simulink model "project"  (R2020a)
settings: Solver=VariableStepAuto  StartTime=0.0  StopTime=1000  RelTol=1e-3
values from neighbouring files (symbols this model uses):
  a = (6371+h)*1e3    (= 6871000)    [AMM_main.m]    (also in Data.m)
  A_RW = sqrt([prop1;prop2;prop3]/(prop1+prop2+prop3))    [AMM_main.m]    (also in Data.m)
  A_t = [Ax;Ay;Az;Ax;Ay;Az;A_sp;A_sp;A_sp;A_sp;]    [AMM_main.m]    (also in Data.m)
  alpha = 0.005    [AMM_main.m]    (also in Data.m = 0.5)
  cd = 2.2    [AMM_main.m]    (also in Data.m)
  horiz_ang_err = rand(3,1) - 0.5    [Data.m]
  horiz_err = 0.25*pi/180    (= 0.00436332312999)    [Data.m]
  init_DCM = DCM0_track    [AMM_main.m]    (also in Data.m = [0.097540404999410   0.957506835434298   0.970592781760616)
  init_orb = orb0_track    [AMM_main.m]    (also in Data.m = [e0,i0,O0,o0,th0])
  init_tumbl = w0_track    [AMM_main.m]    (also in Data.m = 10*pi/180*dir)
  Ir = 1e-7    (= 1e-07)    [AMM_main.m]    (also in Data.m)
  Iz = 2e-7    (= 2e-07)    [AMM_main.m]    (also in Data.m)
  J = [Jx;Jy;Jz]    [AMM_main.m]    (also in Data.m)
  K1 = .05    (= 0.05)    [AMM_main.m]    (also in Data.m)
  K2 = 0.5*K1^2    (= 0.00125)    [AMM_main.m]    (also in Data.m)
  magn_ang_err = rand(3,1) - 0.5    [Data.m]
  magn_err = 2*pi/180    (= 0.0349065850399)    [Data.m]
  max_mx = 1.19    [AMM_main.m]    (also in Data.m)
  max_my = 1.19    [AMM_main.m]    (also in Data.m)
  max_mz = 1.19    [AMM_main.m]    (also in Data.m)
  MS_freq = 1    [AMM_main.m]    (also in Data.m)
  mu = 3.986004418e14    (= 398600441800000)    [AMM_main.m]    (also in Data.m)
  n = sqrt( mu / a^3 )    [AMM_main.m]    (also in Data.m)
  rho = [rho_sMB;rho_dMB;rho_sSP;rho_dSP]    [AMM_main.m]    (also in Data.m)
  rho_air = 4.39e-16 * 1e6/1e3    (= 4.39e-13)    [AMM_main.m]    (also in Data.m)
  RW_Ir = 3.4e-4    (= 0.00034)    [AMM_main.m]    (also in Data.m)
  RW_max_momentum = 400e-3    (= 0.4)    [AMM_main.m]    (also in Data.m)
  RW_max_torque = 100e-3    (= 0.1)    [AMM_main.m]    (also in Data.m)
  wr = 100*pi/180    (= 1.74532925199)    [AMM_main.m]    (also in Data.m)
  ww_earth = 2*pi/(24*3600)*[0;0;1]    [AMM_main.m]    (also in Data.m)
libraries: vrlib x6, simulink x5, dspmtrx3 x2
(part 2 of 2)

== matlab function project/reference DCM/s//c position for a given orbit/Earth's position ==
  data: a input; orb_elements input; r_N output; v_N output
function [r_N,v_N]  = Earth_pos(a,orb_elements)

mu = 3.986004418e14;

e_mod = orb_elements(1);
i     = orb_elements(2);
Omega = orb_elements(3);
omega = orb_elements(4);
theta = orb_elements(5);


h_mod = sqrt(mu*a*(1-e_mod^2));
    
e_unit = rotation_matrix_R3(-Omega) * ...
         rotation_matrix_R1(-i) * ...
         rotation_matrix_R3(-omega) * [1;0;0];
p_unit = rotation_matrix_R3(-Omega) * ...
         rotation_matrix_R1(-i) * ...
         rotation_matrix_R3(-omega) * [0;1;0];
     
r_mod_0 = h_mod^2/mu/(1+e_mod*cos(theta));
r_N       = r_mod_0 * ( cos(theta) * e_unit  +  sin(theta) * p_unit );
v_r     = mu/h_mod * e_mod*sin(theta);
v_theta = mu/h_mod * (1 + e_mod*cos(theta));
v_N       = v_r     * (  cos(theta) * e_unit  +  sin(theta) * p_unit )+ ...
          v_theta * ( -sin(theta) * e_unit  +  cos(theta) * p_unit );
end


function R1 = rotation_matrix_R1(alpha)
%{
rotation_matrix_R1: computes rotation matrix of angle alpha around x axis

INPUT:
	alpha[1]                Angle rotated
                                [rad]

OUTPUT:
    R1 [3x3]                Rotation matrix
                                [(3x3) x -]
%}

R1 = zeros(3);

R1(1,1) = 1;
R1(2,2) =  cos(alpha);
R1(2,3) =  sin(alpha);
R1(3,2) = -sin(alpha);
R1(3,3) =  cos(alpha);
end


function R3 = rotation_matrix_R3(alpha)
%{
rotation_matrix_R3: computes rotation matrix of angle alpha around z axis

INPUT:
	alpha[1]                Angle rotated
                                [rad]

OUTPUT:
    R3 [3x3]                Rotation matrix
                                [(3x3) x -]

%}

R3 = zeros(3);

R3(1,1) =  cos(alpha);
R3(1,2) =  sin(alpha);
R3(2,1) = -sin(alpha);
R3(2,2) =  cos(alpha);
R3(3,3) =  1;
end

== matlab function project/reference DCM/s//c position for a given orbit/orb_elements dynamics/sat motion ==
  data: a input; orb_elements input; orb_elements_dot output
function orb_elements_dot = orbit(a,orb_elements)

mu = 3.986004418e14;

e     = orb_elements(1);
i     = orb_elements(2);
O = orb_elements(3);
o = orb_elements(4);
theta = orb_elements(5); %true anomaly


n     = sqrt( mu / a^3 ); %mean motion: angular speed required to complete 1 orbit

orb_elements_dot    = zeros (size(orb_elements));

orb_elements_dot(5) = n * (1 + e*cos(theta))^2 / (1 - e^2)^(3/2);

== matlab function project/Sun direction wrt s//c body frame/Sun's direction ==
  data: t input; S_N output
function S_N = fcn(t)

%% data
Rs = 149597870700; %[m] but we can substitute it by 1 so we have a unitary vector
Rs = 1;
epsilon = 23.45 * pi/180; %[rad]
T = 365.25*24*3600; %[s]
nsun = 2*pi/T; % [s^-1]

%% 
S_N = Rs * [cos(nsun*t);
            sin(nsun*t)*cos(epsilon);
            sin(nsun*t)*sin(epsilon);];

end

== matlab function project/magnetic torquer detumbling control/magn.vector body frame/Magnetic model ==
  data: r_N input; b_N output; t input
function b_N = fcn(r_N,t)
% coefficients
IGRF = '2000';
switch IGRF
    case '1995'
        g0_1 = -29682e-9;
        g1_1 = -1789e-9;
        h1_1 = 5318e-9;
    case '2000'
        g0_1 = -29615e-9;
        g1_1 = -1728e-9;
        h1_1 = 5186e-9;
end


w = 360/(24*3600) * pi/180; %[rad/s] angular rotation speed of Earth
decl = 11.5*pi/180; %[rad]
R = 6371.2e3; %equatorial radius [m]
r = norm(r_N);
rr_unit = r_N/r; %unitary vector

H0 = sqrt(g0_1^2 + g1_1^2 + h1_1^2);
m = [
    sin(decl)*cos(w*t);
    sin(decl)*sin(w*t);
    cos(decl)
    ]; %unit vector along dipole axis

b_N = R^3*H0/r^3*(3*(dot(m,rr_unit))*rr_unit - m); %Earth's MF in the inertial frame

== matlab function project/magnetic torquer detumbling control/magn.vector body frame/s//c position for a given orbit/Earth's position ==
  data: a input; orb_elements input; r_N output; v_N output
function [r_N,v_N]  = Earth_pos(a,orb_elements)

mu = 3.986004418e14;

e_mod = orb_elements(1);
i     = orb_elements(2);
Omega = orb_elements(3);
omega = orb_elements(4);
theta = orb_elements(5);


h_mod = sqrt(mu*a*(1-e_mod^2));
    
e_unit = rotation_matrix_R3(-Omega) * ...
         rotation_matrix_R1(-i) * ...
         rotation_matrix_R3(-omega) * [1;0;0];
p_unit = rotation_matrix_R3(-Omega) * ...
         rotation_matrix_R1(-i) * ...
         rotation_matrix_R3(-omega) * [0;1;0];
     
r_mod_0 = h_mod^2/mu/(1+e_mod*cos(theta));
r_N       = r_mod_0 * ( cos(theta) * e_unit  +  sin(theta) * p_unit );
v_r     = mu/h_mod * e_mod*sin(theta);
v_theta = mu/h_mod * (1 + e_mod*cos(theta));
v_N       = v_r     * (  cos(theta) * e_unit  +  sin(theta) * p_unit )+ ...
          v_theta * ( -sin(theta) * e_unit  +  cos(theta) * p_unit );
end


function R1 = rotation_matrix_R1(alpha)
%{
rotation_matrix_R1: computes rotation matrix of angle alpha around x axis

INPUT:
	alpha[1]                Angle rotated
                                [rad]

OUTPUT:
    R1 [3x3]                Rotation matrix
                                [(3x3) x -]
%}

R1 = zeros(3);

R1(1,1) = 1;
R1(2,2) =  cos(alpha);
R1(2,3) =  sin(alpha);
R1(3,2) = -sin(alpha);
R1(3,3) =  cos(alpha);
end


function R3 = rotation_matrix_R3(alpha)
%{
rotation_matrix_R3: computes rotation matrix of angle alpha around z axis

INPUT:
	alpha[1]                Angle rotated
                                [rad]

OUTPUT:
    R3 [3x3]                Rotation matrix
                                [(3x3) x -]

%}

R3 = zeros(3);

R3(1,1) =  cos(alpha);
R3(1,2) =  sin(alpha);
R3(2,1) = -sin(alpha);
R3(2,2) =  cos(alpha);
R3(3,3) =  1;
end

== matlab function project/Disturbances: -grav.gradient -airdrag -SRP -magnetic field/magnetic torque/magnetic model/Magnetic model ==
  data: r_N input; b_N output; t input
function b_N = fcn(r_N,t)
% coefficients
IGRF = '2000';
switch IGRF
    case '1995'
        g0_1 = -29682e-9;
        g1_1 = -1789e-9;
        h1_1 = 5318e-9;
    case '2000'
        g0_1 = -29615e-9;
        g1_1 = -1728e-9;
        h1_1 = 5186e-9;
end


w = 360/(24*3600) * pi/180; %[rad/s] angular rotation speed of Earth
decl = 11.5*pi/180; %[rad]
R = 6371.2e3; %equatorial radius [m]
r = norm(r_N);
rr_unit = r_N/r; %unitary vector

H0 = sqrt(g0_1^2 + g1_1^2 + h1_1^2);
m = [
    sin(decl)*cos(w*t);
    sin(decl)*sin(w*t);
    cos(decl)
    ]; %unit vector along dipole axis

b_N = R^3*H0/r^3*(3*(dot(m,rr_unit))*rr_unit - m); %Earth's MF in the inertial frame

== matlab function project/Disturbances: -grav.gradient -airdrag -SRP -magnetic field/magnetic torque/magnetic model/s//c position for a given orbit/Earth's position ==
  data: a input; orb_elements input; r_N output; v_N output
function [r_N,v_N]  = Earth_pos(a,orb_elements)

mu = 3.986004418e14;

e_mod = orb_elements(1);
i     = orb_elements(2);
Omega = orb_elements(3);
omega = orb_elements(4);
theta = orb_elements(5);


h_mod = sqrt(mu*a*(1-e_mod^2));
    
e_unit = rotation_matrix_R3(-Omega) * ...
         rotation_matrix_R1(-i) * ...
         rotation_matrix_R3(-omega) * [1;0;0];
p_unit = rotation_matrix_R3(-Omega) * ...
         rotation_matrix_R1(-i) * ...
         rotation_matrix_R3(-omega) * [0;1;0];
     
r_mod_0 = h_mod^2/mu/(1+e_mod*cos(theta));
r_N       = r_mod_0 * ( cos(theta) * e_unit  +  sin(theta) * p_unit );
v_r     = mu/h_mod * e_mod*sin(theta);
v_theta = mu/h_mod * (1 + e_mod*cos(theta));
v_N       = v_r     * (  cos(theta) * e_unit  +  sin(theta) * p_unit )+ ...
          v_theta * ( -sin(theta) * e_unit  +  cos(theta) * p_unit );
end


function R1 = rotation_matrix_R1(alpha)
%{
rotation_matrix_R1: computes rotation matrix of angle alpha around x axis

INPUT:
	alpha[1]                Angle rotated
                                [rad]

OUTPUT:
    R1 [3x3]                Rotation matrix
                                [(3x3) x -]
%}

R1 = zeros(3);

R1(1,1) = 1;
R1(2,2) =  cos(alpha);
R1(2,3) =  sin(alpha);
R1(3,2) = -sin(alpha);
R1(3,3) =  cos(alpha);
end


function R3 = rotation_matrix_R3(alpha)
%{
rotation_matrix_R3: computes rotation matrix of angle alpha around z axis

INPUT:
	alpha[1]                Angle rotated
                                [rad]

OUTPUT:
    R3 [3x3]                Rotation matrix
                                [(3x3) x -]

%}

R3 = zeros(3);

R3(1,1) =  cos(alpha);
R3(1,2) =  sin(alpha);
R3(2,1) = -sin(alpha);
R3(2,2) =  cos(alpha);
R3(3,3) =  1;
end

== matlab function project/Disturbances: -grav.gradient -airdrag -SRP -magnetic field/magnetic torque/magnetic model/s//c position for a given orbit/orb_elements dynamics/sat motion ==
  data: a input; orb_elements input; orb_elements_dot output
function orb_elements_dot = orbit(a,orb_elements)

mu = 3.986004418e14;

e     = orb_elements(1);
i     = orb_elements(2);
O = orb_elements(3);
o = orb_elements(4);
theta = orb_elements(5); %true anomaly


n     = sqrt( mu / a^3 ); %mean motion: angular speed required to complete 1 orbit

orb_elements_dot    = zeros (size(orb_elements));

orb_elements_dot(5) = n * (1 + e*cos(theta))^2 / (1 - e^2)^(3/2);

== matlab function project/DCM Kinematics/hat ==
  data: w input; w_hat output
function w_hat = hat_fcn(w)

w_hat       = zeros (3);

w_hat (1,2) = - w(3);
w_hat (1,3) =   w(2);
w_hat (2,1) =   w(3);
w_hat (2,3) = - w(1);
w_hat (3,1) = - w(2);
w_hat (3,2) =   w(1);

== matlab function project/magnetic torquer detumbling control/magn.vector body frame/s//c position for a given orbit/orb_elements dynamics/sat motion ==
  data: a input; orb_elements input; orb_elements_dot output
function orb_elements_dot = orbit(a,orb_elements)

mu = 3.986004418e14;

e     = orb_elements(1);
i     = orb_elements(2);
O = orb_elements(3);
o = orb_elements(4);
theta = orb_elements(5); %true anomaly


n     = sqrt( mu / a^3 ); %mean motion: angular speed required to complete 1 orbit

orb_elements_dot    = zeros (size(orb_elements));

orb_elements_dot(5) = n * (1 + e*cos(theta))^2 / (1 - e^2)^(3/2);

== matlab function project/dynamic equation ==
  data: M input; u input; J input; w input; wdot output
function wdot = fcn(M,u,J,w)
%data
% J1 = 100.9e-2; %[kg m^2]
% J2 =  25.1e-2;
% J3 =  91.6e-2;
J1 = J(1);
J2 = J(2);
J3 = J(3);

% diff equation
wdot = zeros(size(w));

wdot(1) = (J2 - J3)/J1 * w(2) * w(3) + u(1)/J1 + M(1)/J1;
wdot(2) = (J3 - J1)/J2 * w(1) * w(3) + u(2)/J2 + M(2)/J2;
wdot(3) = (J1 - J2)/J3 * w(1) * w(2) + u(3)/J3 + M(3)/J3;

end

== matlab function project/Disturbances: -grav.gradient -airdrag -SRP -magnetic field/SRP moment/SRP disturbance torque ==
  data: S_B input; T_srp output; A input; rho input
function T_srp = fcn(S_B,A,rho)

% Solar Radiation Pressure
F_e = 1358;
c   = 3e8;
P   =  F_e / c;

% Displaced CoM
r_CoM = 1.8e-2 * [1; 0; 0]; %considering x-axis displaced

% SC main body
n = zeros(3,10);
n(:,1) = [1; 0; 0];
n(:,2) = [0; 1; 0];
n(:,3) = [0; 0; 1];
n(:,4) = - n(:,1);
n(:,5) = - n(:,2);
n(:,6) = - n(:,3);

% % Area
% A = zeros(10,1);
% A(1) = 6*0.1*0.1; %s/c area
% A(2) = 4*0.1*0.1;
% A(3) = A(1);
% A(4) = A(1);
% A(5) = A(2);
% A(6) = A(3);
% A(7)  = 5*0.1*0.1; %solar panel area
% A(8)  = A(7);
% A(9)  = A(7);
% A(10) = A(9);

% position of center of pressure of the flat surface wrt the center of mass
r = zeros(3,10);
r(:,1) =  0.1*[1; 0; 0] - r_CoM; %typical CoP locations
r(:,2) = 0.15*[0; 1; 0] - r_CoM; %typical CoP locations
r(:,3) =  0.1*[0; 0; 1] - r_CoM; %typical CoP locations
r(:,4) = - r(:,1) - r_CoM;
r(:,5) = - r(:,2) - r_CoM;
r(:,6) = - r(:,3) - r_CoM;

rho_sMB = rho(1);
rho_dMB = rho(2);

% SC solar panels
n(:,7)  =   n(:,1);
n(:,8)  = - n(:,1);
n(:,9)  =   n(:,2);
n(:,10) = - n(:,2);

r(:,7)  =  0.25*[0; 0; 1] - r_CoM;
r(:,8)  =  r(:,7);
r(:,9)  = -0.25*[0; 0; 1] - r_CoM;
r(:,10) =  r(:,9);

rho_sSP = rho(3);
rho_dSP = rho(4);

% Forces on each side and resulting torque
F = zeros(3,10);
for i = 1:6
    if dot(S_B,n(:,i)) > 0
        F(:,i) = - P * A(i) * dot(S_B,n(:,i)) * ...
           (  (1-rho_sMB)*S_B +         ...
             ( 2*rho_sMB*dot(S_B,n(:,i)) + 2/3*rho_dMB) * n(:,i) );
    else
        F(:,i) = [0;0;0];
    end
end

for i = 7:10
    if dot(S_B,n(:,i)) > 0
        F(:,i) = - P * A(i) * dot(S_B,n(:,i)) * ...
           (  (1-rho_sSP)*S_B +         ...
             ( 2*rho_sSP*dot(S_B,n(:,i)) + 2/3*rho_dSP) * n(:,i) );
    else
        F(:,i) = [0;0;0];
    end
end

T_srp = zeros(3,1);
for i=length(F)
    T_srp = T_srp + cross(r(:,i),F(:,i));
end

end %function

== matlab function project/Disturbances: -grav.gradient -airdrag -SRP -magnetic field/air drag/air drag ==
  data: vv_r input; M_drag output; A input; rho input; cd input
function M_drag = fcn(vv_r,A,rho,cd)

v_r = norm(vv_r); % 
% rho = 4.39e-16 * 1e6/1e3; %[kg/m3] rho density at constant altitude 500km
% cd = 2.2; %typical value

% Displaced CoM
r_CoM = 1.8e-2 * [1; 0; 0]; %considering x-axis displaced

% SC main body
n = zeros(3,10);
n(:,1) = [1; 0; 0];
n(:,2) = [0; 1; 0];
n(:,3) = [0; 0; 1];
n(:,4) = - n(:,1);
n(:,5) = - n(:,2);
n(:,6) = - n(:,3);
% SC solar panels
n(:,7)  =   n(:,1);
n(:,8)  = - n(:,1);
n(:,9)  =   n(:,2);
n(:,10) = - n(:,2);

% Area
% A = zeros(10,1);
% A(1) = 6*0.1*0.1;
% A(2) = 4*0.1*0.1;
% A(3) = A(1);
% A(4) = A(1);
% A(5) = A(2);
% A(6) = A(3);
% A(7)  = 5*0.1*0.1;
% A(8)  = A(7);
% A(9)  = A(7);
% A(10) = A(9);

% r: position vector from s/c CoM to CoP of surface Ai
r = zeros(3,10);
r(:,1) =  0.1*[1; 0; 0] - r_CoM; %typical CoP locations
r(:,2) = 0.15*[0; 1; 0] - r_CoM; %typical CoP locations
r(:,3) =  0.1*[0; 0; 1] - r_CoM; %typical CoP locations
r(:,4) = - r(:,1) - r_CoM;
r(:,5) = - r(:,2) - r_CoM;
r(:,6) = - r(:,3) - r_CoM;
r(:,7)  =  0.25*[0; 0; 1] - r_CoM;
r(:,8)  =  r(:,7);
r(:,9)  = -0.25*[0; 0; 1] - r_CoM;
r(:,10) =  r(:,9);

F = zeros(3,10);
M_drag = zeros(3,1);
for i=1:10
    if dot(n(:,i),vv_r/v_r) > 0
        F(:,i) = -0.5*cd*rho*v_r^2*A(i)*vv_r/v_r*dot(n(:,i),vv_r/v_r);
    end
    M_drag = M_drag + cross(r(:,i),F(:,i));
end

end %function

== matlab function project/Disturbances: -grav.gradient -airdrag -SRP -magnetic field/air drag/s//c position for a given orbit/Earth's position ==
  data: a input; orb_elements input; r_N output; v_N output
function [r_N,v_N]  = Earth_pos(a,orb_elements)

mu = 3.986004418e14;

e_mod = orb_elements(1);
i     = orb_elements(2);
Omega = orb_elements(3);
omega = orb_elements(4);
theta = orb_elements(5);


h_mod = sqrt(mu*a*(1-e_mod^2));
    
e_unit = rotation_matrix_R3(-Omega) * ...
         rotation_matrix_R1(-i) * ...
         rotation_matrix_R3(-omega) * [1;0;0];
p_unit = rotation_matrix_R3(-Omega) * ...
         rotation_matrix_R1(-i) * ...
         rotation_matrix_R3(-omega) * [0;1;0];
     
r_mod_0 = h_mod^2/mu/(1+e_mod*cos(theta));
r_N       = r_mod_0 * ( cos(theta) * e_unit  +  sin(theta) * p_unit );
v_r     = mu/h_mod * e_mod*sin(theta);
v_theta = mu/h_mod * (1 + e_mod*cos(theta));
v_N       = v_r     * (  cos(theta) * e_unit  +  sin(theta) * p_unit )+ ...
          v_theta * ( -sin(theta) * e_unit  +  cos(theta) * p_unit );
end


function R1 = rotation_matrix_R1(alpha)
%{
rotation_matrix_R1: computes rotation matrix of angle alpha around x axis

INPUT:
	alpha[1]                Angle rotated
                                [rad]

OUTPUT:
    R1 [3x3]                Rotation matrix
                                [(3x3) x -]
%}

R1 = zeros(3);

R1(1,1) = 1;
R1(2,2) =  cos(alpha);
R1(2,3) =  sin(alpha);
R1(3,2) = -sin(alpha);
R1(3,3) =  cos(alpha);
end


function R3 = rotation_matrix_R3(alpha)
%{
rotation_matrix_R3: computes rotation matrix of angle alpha around z axis

INPUT:
	alpha[1]                Angle rotated
                                [rad]

OUTPUT:
    R3 [3x3]                Rotation matrix
                                [(3x3) x -]

%}

R3 = zeros(3);

R3(1,1) =  cos(alpha);
R3(1,2) =  sin(alpha);
R3(2,1) = -sin(alpha);
R3(2,2) =  cos(alpha);
R3(3,3) =  1;
end

== matlab function project/Disturbances: -grav.gradient -airdrag -SRP -magnetic field/air drag/s//c position for a given orbit/orb_elements dynamics/sat motion ==
  data: a input; orb_elements input; orb_elements_dot output
function orb_elements_dot = orbit(a,orb_elements)

mu = 3.986004418e14;

e     = orb_elements(1);
i     = orb_elements(2);
O = orb_elements(3);
o = orb_elements(4);
theta = orb_elements(5); %true anomaly


n     = sqrt( mu / a^3 ); %mean motion: angular speed required to complete 1 orbit

orb_elements_dot    = zeros (size(orb_elements));

orb_elements_dot(5) = n * (1 + e*cos(theta))^2 / (1 - e^2)^(3/2);

== matlab function project/DCM feedback control/DCM feedback ==
  data: w input; A_e input; K1 input; K2 input; u output; J input; mu input; a input
function u = DCM_fbk_control(w,A_e,K1,K2,J,mu,a)


w_ref = [0; 0; -sqrt(mu/a^3) ];
I_x = J(1);
I_y = J(2);
I_z = J(3);

% u = -K1*w - K2*[A_e(2,3)-A_e(3,2); A_e(3,1)-A_e(1,3); A_e(1,2)-A_e(2,1)];
u = - K1 * [I_x;I_y;I_z].*(w - w_ref) ...
    - K2 * [I_x;I_y;I_z].*[A_e(2,3)-A_e(3,2); A_e(3,1)-A_e(1,3); A_e(1,2)-A_e(2,1)] ...
    + cross ( w, [I_x;I_y;I_z].*w );
%     - K3 * sign(w) ...
%     + K2 * ( (trace(A_e)-1)*[A_e(3,2)-A_e(2,3); A_e(1,3)-A_e(3,1); A_e(2,1)-A_e(1,2)] - w ) ...

% Avoid excesive rotational rate problematic for attitude acquisition (0.5 deg/s)
u_sat_max = - K1 * [I_x;I_y;I_z].*(w - 0.45*pi/180*[1;1;1]/sqrt(3)) ...
            + cross ( w, [I_x;I_y;I_z].*w );
u_sat_min = - K1 * [I_x;I_y;I_z].*(w + 0.45*pi/180*[1;1;1]/sqrt(3)) ...
            + cross ( w, [I_x;I_y;I_z].*w );
for i = 1:3
    if ( u(i)*w(i) > 0 ) && ( abs(w(i)) > 0.4*pi/180/sqrt(3) )
%         u(i) = - K1*w(i);
%         u(i) = - K1*sign(w(i))*(abs(w(i)) - 0.45*pi/180);
        if w(i)>0
            u(i) = u_sat_max(i);
        else
            u(i) = u_sat_min(i);
        end
    end
end
end

== matlab function project/magnetic torquer detumbling control/ideal control law ==
  data: M input; b input; m output
function m = fcn(M,b)

m = cross(b,M)./b.^2;
